simulink model "Beobachter"  (Simulink 7.9)
settings: Solver=ode45  StartTime=0.0  StopTime=4  RelTol=1e-3
values from neighbouring files (symbols this model uses):
  bias = 1    [init.m]
  l_1 = 8.    (= 8)    [init.m]
  l_2 = 15.18    [init.m]
  l_3 = 25.45    [init.m]
undefined symbols (not defined in the file or in its folder): sigbuilder_block
libraries: simulink x2
settings Model: Creator=Matthias  LastModifiedBy=Matthias

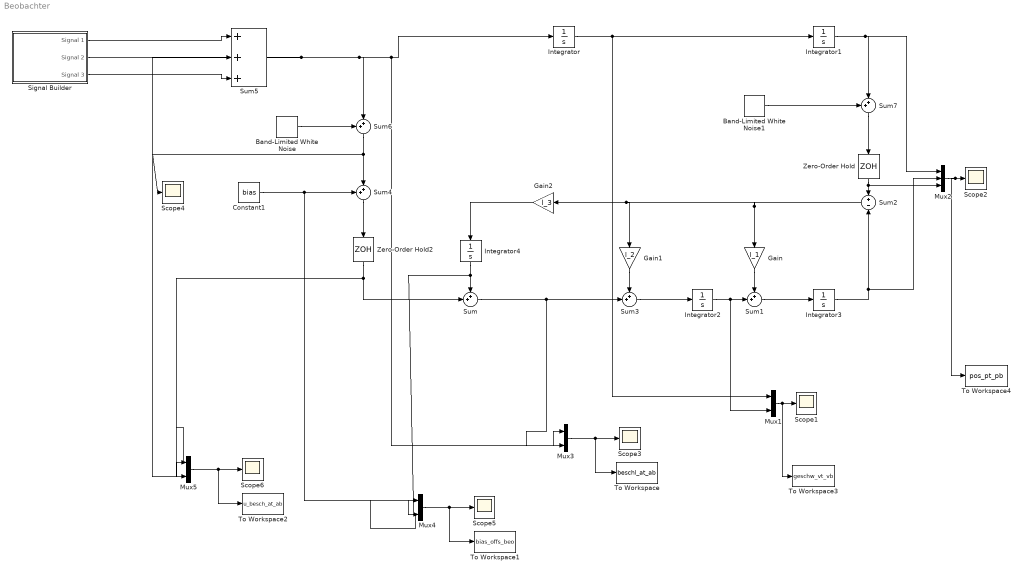
== system Beobachter ==
  Band-Limited White Noise : simulink/Sources/Band-Limited White Noise  Cov=[0.00001]  Ts=0.001  seed=[23341]
  Band-Limited White Noise1 : simulink/Sources/Band-Limited White Noise  Cov=[0.0001]  Ts=0.025  seed=[23341]
  Constant1 : Constant  Value=bias
  Gain : Gain  Gain=l_1
  Gain1 : Gain  Gain=l_2
  Gain2 : Gain  Gain=l_3
  Integrator{,1..4} (5 alike) : Integrator
  Mux{1,3..5} (4 alike) : Mux  Inputs=2
  Mux2 : Mux  Inputs=3
  Scope{1..6} (6 alike) : Scope
      Scope2 settings: SaveName=ScopeData2
      Scope3 settings: SaveName=ScopeData3
      Scope4 settings: SaveName=ScopeData4
      Scope6 settings: SaveName=ScopeData5
  Signal Builder : Subsystem  Tag=STV Subsys  LoadFcn=sigbuilder_block('load',[403.5 141 550.5 395.25 ]);  StartFcn=sigbuilder_block('start');  StopFcn=sigbuilder_block('stop');  ClipboardFcn=sigbuilder_block('clipboard');  mask(Sigbuilder block){}
      mask help: Simulink:masks:SigbuilderBlock_MD
      mask init:
      | if ~strcmp(get_param(bdroot(gcbh),'SimulationStatus'),'stopped') tuvar = sigbuilder_block('maskInit'); end
      settings: CopyFcn=sigbuilder_block('copy');  DeleteFcn=sigbuilder_block('delete');  ModelCloseFcn=sigbuilder_block('modelClose');  PreSaveFcn=sigbuilder_block('preSave');  PauseFcn=sigbuilder_block('pause');  ContinueFcn=sigbuilder_block('continue');  NameChangeFcn=sigbuilder_block('namechange');  OpenFcn=sigbuilder_block('open',[437.6 199.2 550.4 400 ]);  CloseFcn=sigbuilder_block('close');
      mask Display: plot(0, 0, 100, 100,[2, 2, 32, 32, 2], [68, 8, 8, 68, 68],[32, 2], [38, 38], [32, 19, 2],[53, 60, 44], [32, 17, 17, 2],[16, 16, 31, 31]);txt = getActiveGroup(gcbh);text(2, 100, txt,'verticalAlignment', 'top');
  Sum{,1,3..4,6..7} (6 alike) : Sum  Inputs=++|
  Sum2 : Sum  Inputs=+|-
  Sum5 : Sum  Inputs=+++
  To Workspace : ToWorkspace  VariableName=beschl_at_ab  SampleTime=-1  SaveFormat=Structure With Time
  To Workspace1 : ToWorkspace  VariableName=bias_offs_beo  SampleTime=-1  SaveFormat=Structure With Time
  To Workspace2 : ToWorkspace  VariableName=u_besch_at_ab  SampleTime=-1  SaveFormat=Structure With Time
  To Workspace3 : ToWorkspace  VariableName=geschw_vt_vb  SampleTime=-1  SaveFormat=Structure With Time
  To Workspace4 : ToWorkspace  VariableName=pos_pt_pb  SampleTime=-1  SaveFormat=Structure With Time
  Zero-Order Hold : ZeroOrderHold  SampleTime=.025
  Zero-Order Hold2 : ZeroOrderHold  SampleTime=.001
  wires:
  Integrator2/1 -> Sum1/2, Mux1/2
  Sum1/1 -> Integrator3/1
  Integrator1/1 -> Mux2/1, Sum7/2
  Integrator3/1 -> Sum2/2, Mux2/2
  Gain/1 -> Sum1/1
  Sum2/1 -> Gain/1, Gain2/1, Gain1/1
  Sum3/1 -> Integrator2/1
  Gain1/1 -> Sum3/1
  Integrator4/1 -> Sum/1, Mux4/2
  Sum/1 -> Sum3/2, Mux3/2
  Gain2/1 -> Integrator4/1
  Integrator/1 -> Integrator1/1, Mux1/1
  Constant1/1 -> Sum4/1, Mux4/1
  Sum4/1 -> Zero-Order Hold2/1
  Mux1/1 -> Scope1/1, To Workspace3/1
  Mux2/1 -> Scope2/1, To Workspace4/1
  Mux3/1 -> Scope3/1, To Workspace/1
  Zero-Order Hold/1 -> Sum2/1, Mux2/3
  Zero-Order Hold2/1 -> Sum/2, Mux5/2
  Signal Builder/1(Signal 1) -> Sum5/1
  Signal Builder/2(Signal 2) -> Sum5/2
  Sum5/1 -> Integrator/1, Mux3/1, Sum6/2, Mux5/1
  Signal Builder/3(Signal 3) -> Sum5/3
  Sum6/1 -> Sum4/2, Scope4/1
  Band-Limited White Noise/1 -> Sum6/1
  Sum7/1 -> Zero-Order Hold/1
  Band-Limited White Noise1/1 -> Sum7/1
  Mux4/1 -> To Workspace1/1, Scope5/1
  Mux5/1 -> To Workspace2/1, Scope6/1

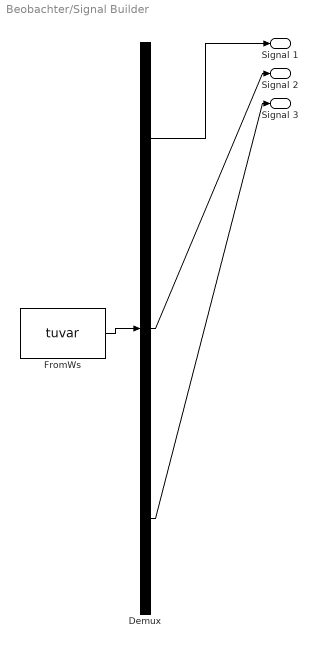
== system Beobachter/Signal Builder ==
  Demux : Demux  Tag=STV Demux  Outputs=3
  FromWs : FromWorkspace  Tag=STV FromWs  VariableName=tuvar  SampleTime=0  SigBuilderData=DataTag0  VnvData=DataTag1
      SigBuilderData=|
      | common.afterFinalStr = 'Extrapolate'
      | common.sampleTime = 0
      | dataSet.timeRange = [0 10]
      | dataSet.name = 'Group 1'
      | sbobj.Groups.Name = 'Group 1'
      | sbobj.Groups.Signals(1).Name = 'Signal 1'
      | sbobj.Groups.Signals(1).XData = [0 2 2.2 2.8 3 10]
      | sbobj.Groups.Signals(1).YData = [0 0 -3 -4 0 0]
      | sbobj.Groups.Signals(2).Name = 'Signal 2'
      | sbobj.Groups.Signals(2).XData = [0 6 6.5 7 7.5 10]
      | sbobj.Groups.Signals(2).YData = [0 0 -9.8 -10 0 0]
      | sbobj.Groups.Signals(3).Name = 'Signal 3'
      | sbobj.Groups.Signals(3).XData = [0 3.2 3.3 3.8 6.5 10]
      | sbobj.Groups.Signals(3).YData = [0 0 15.5 0 0 0]
  Signal 1 : Outport  Tag=STV Outport
  Signal 2 : Outport  Tag=STV Outport  Port=2
  Signal 3 : Outport  Tag=STV Outport  Port=3
  wires:
  Demux/1 -> Signal 1/1
  FromWs/1 -> Demux/1
  Demux/2 -> Signal 2/1
  Demux/3 -> Signal 3/1
